simulink model "interp_compare_1d_R2019a"  (R2019a)
settings: Solver=FixedStepDiscrete  StartTime=0.0  StopTime=1  FixedStep=1  RelTol=1e-3
Description:
  | 1-D Lagrange vs Linear point-slope (Prelookup path)
settings Model: Creator=Administrator  LastModifiedBy=Administrator
settings DebuggingCC: UnconnectedInputMsg=none  UnconnectedOutputMsg=none  UnconnectedLineMsg=none
settings ModelReferenceCC: UpdateModelReferenceTargets=IfOutOfDate  EnableRefExpFcnMdlSchedulingChecks=off
settings RTWCC: Description=Generic Real-Time Target
settings ConfigComp: CovBoundaryAbsTol=1.0e-5

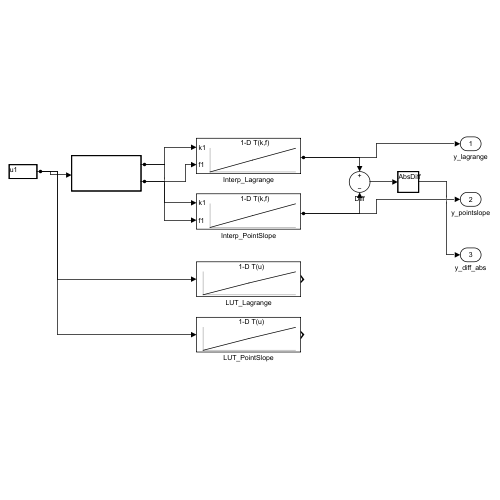
[thumbnail: Simulink's stored preview of the top-level diagram]
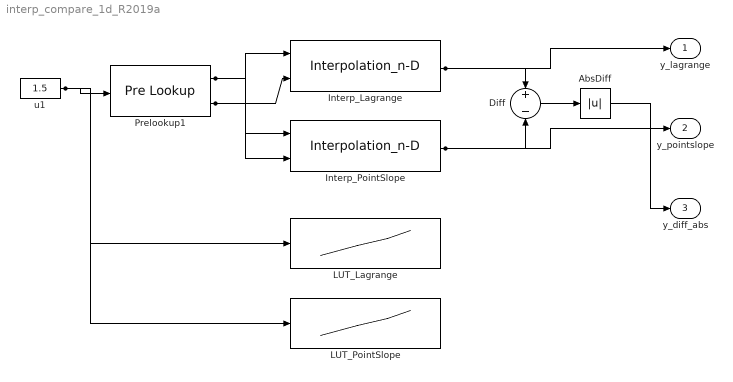
== system interp_compare_1d_R2019a ==
  AbsDiff : Abs
  Diff : Sum  Inputs=+-
  Interp_Lagrange : Interpolation_n-D  NumberOfTableDimensions=1  Table=[200;500;800]  InterpMethod=Linear Lagrange  ExtrapMethod=Clip  InternalRulePriority=Speed
      settings: InputPortMap=u0,u1
  Interp_PointSlope : Interpolation_n-D  NumberOfTableDimensions=1  Table=[200;500;800]  ExtrapMethod=Clip  InternalRulePriority=Speed
      settings: InputPortMap=u0,u1
  LUT_Lagrange : Lookup_n-D  NumberOfTableDimensions=1  BreakpointsForDimension1=[1 2 3]  Table=[200;500;800]  InterpMethod=Linear Lagrange  ExtrapMethod=Clip  InternalRulePriority=Speed  RndMeth=Simplest  InputSameDT=on
  LUT_PointSlope : Lookup_n-D  NumberOfTableDimensions=1  BreakpointsForDimension1=[1 2 3]  Table=[200;500;800]  ExtrapMethod=Clip  InternalRulePriority=Speed  RndMeth=Simplest  InputSameDT=on
  Prelookup1 : PreLookup  BreakpointsData=[1 2 3]
  u1 : Constant  Value=1.5
  y_lagrange : Outport
  y_pointslope : Outport  Port=2
  y_diff_abs : Outport  Port=3
  wires:
  u1/1 -> Prelookup1/1, LUT_Lagrange/1, LUT_PointSlope/1
  Prelookup1/1 -> Interp_Lagrange/1, Interp_PointSlope/1
  Prelookup1/2 -> Interp_Lagrange/2, Interp_PointSlope/2
  Interp_Lagrange/1 -> Diff/1, y_lagrange/1
  Interp_PointSlope/1 -> Diff/2, y_pointslope/1
  Diff/1 -> AbsDiff/1
  AbsDiff/1 -> y_diff_abs/1
